simulink model "part 2 - overshootandsettlingtime"  (R2024b)
settings: Solver=VariableStepAuto  StartTime=0.0  StopTime=0.1  MaxStep=1e-6  RelTol=1e-3
values from neighbouring files (symbols this model uses):
  C = delta_iL / (fs * delta_Uc * 8)    (= 0.000625)    [part2 - overshootandsettlingtime.m]    (also in projectpart4.m; projectpart5.m)
  L = ((Uin - Uout) * u) / (delta_iL * fs)    (= 0.0028125)    [part2 - overshootandsettlingtime.m]    (also in projectpart4.m; projectpart5.m)
  R = Uout / Iout_max    (= 1.8)    [part2 - overshootandsettlingtime.m]    (also in projectpart4.m; projectpart5.m)
settings Model: Creator=Talida  LastModifiedBy=Talida

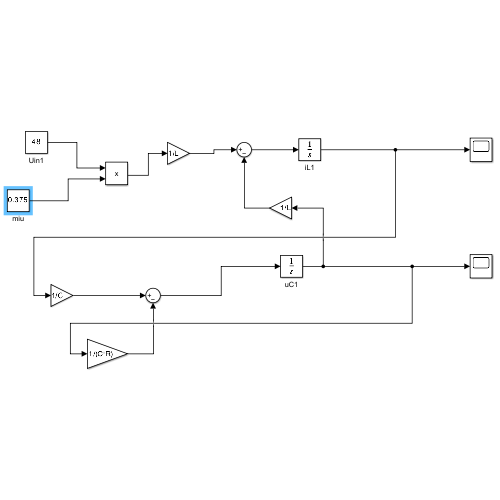
[thumbnail: Simulink's stored preview of the top-level diagram]
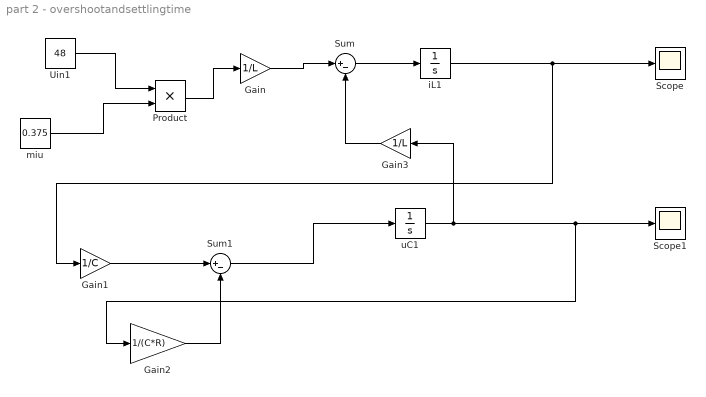
== system part 2 - overshootandsettlingtime ==
  Gain : Gain  Gain=1/L
  Gain1 : Gain  Gain=1/C
  Gain2 : Gain  Gain=1/(C*R)
  Gain3 : Gain  Gain=1/L
  Product : Product
  Scope : Scope
  Scope1 : Scope
  Sum : Sum  Inputs=|+-
  Sum1 : Sum  Inputs=|+-
  Uin1 : Constant  Value=48
  iL1 : Integrator
  miu : Constant  Value=0.375
  uC1 : Integrator
  wires:
  Gain1/1 -> Sum1/1
  Sum/1 -> iL1/1
  iL1/1 -> Gain1/1, Scope/1
  uC1/1 -> Gain3/1, Gain2/1, Scope1/1
  Gain3/1 -> Sum/2
  Gain/1 -> Sum/1
  Sum1/1 -> uC1/1
  Uin1/1 -> Product/1
  miu/1 -> Product/2
  Product/1 -> Gain/1
  Gain2/1 -> Sum1/2
